simulink model "IEEE9_16b_forward"  (R2020a)
settings: Solver=VariableStepAuto  StartTime=0.0  StopTime=5  MaxStep=1e-4  RelTol=1e-3
libraries: powerlib x33, dspsigops x6, sps_avr x3
(part 1 of 2)
settings Model: Creator=Pankaj  LastModifiedBy=ahmed
settings DataIOCC: ReturnWorkspaceOutputs=off
settings DebuggingCC: UnconnectedInputMsg=none  UnconnectedOutputMsg=none  UnconnectedLineMsg=none  ArithmeticOperatorsInVariantConditions=warning
settings SFSimCC: SimUseLocalCustomCode=off  CustomCodeUndefinedFunction=UseInterfaceOnly
settings RTWCC: RTWUseLocalCustomCode=off
settings CodeAppCC: StateflowObjectComments=on
settings SimscapeCC: SimscapeNormalizeSystem=off

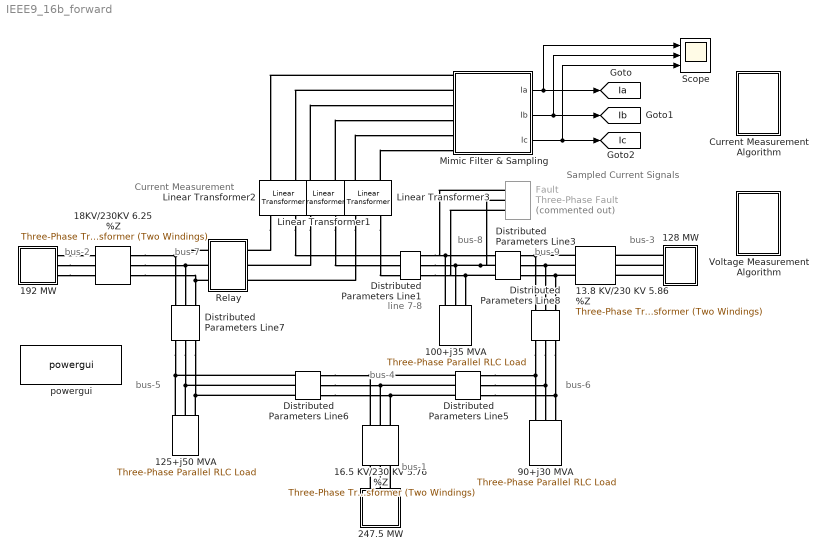
== system IEEE9_16b_forward ==
  note: Current Measurement
  note: Sampled Current Signals
  note: bus-2
  note: bus-7
  note: bus-8
  note: bus-9
  note: bus-1
  note: bus-3
  note: bus-4
  note: bus-6
  note: bus-5
  note: line 7-8
  100+j35 MVA : powerlib/Elements/Three-Phase Parallel RLC Load  LConnTagsString=A|B|C  Configuration=Y (grounded)  NominalVoltage=(230000)*0.993698  Vabc=[1e3 1e3 1e3]  Vabcp=[1e3 1e3 1e3]  NominalFrequency=60  UnbalancedPower=off  ActivePower=100e6  InductivePower=35e6  CapacitivePower=0  Pabc=[10e3 9e3 11e3]  QLabc=[100 90 110]  QCabc=[100 90 110]  Pabcp=[10e3 9e3 11e3]  QLabcp=[100 90 110]  QCabcp=[100 90 110]  Measurements=None  LoadType=constant PQ
  125+j50 MVA : powerlib/Elements/Three-Phase Parallel RLC Load  LConnTagsString=A|B|C  Configuration=Y (grounded)  NominalVoltage=(223027)*1  Vabc=[1e3 1e3 1e3]  Vabcp=[1e3 1e3 1e3]  NominalFrequency=60  UnbalancedPower=off  ActivePower=125e6  InductivePower=50e6  CapacitivePower=0  Pabc=[10e3 9e3 11e3]  QLabc=[100 90 110]  QCabc=[100 90 110]  Pabcp=[10e3 9e3 11e3]  QLabcp=[100 90 110]  QCabcp=[100 90 110]  Measurements=None  LoadType=constant PQ
  128 MW : Subsystem
  13.8 KV/230 KV 5.86 %Z : powerlib/Elements/Three-Phase Transformer (Two Windings)  Winding1Connection=Yg  Winding2Connection=Yg  CoreType=Three single-phase transformers  SetSaturation=off  Hysteresis=off  DataFile='hysteresis'  SetInitialFlux=off  Measurements=None  UNITS=pu  NominalPower=[ 100e6 , 60 ]  Winding1=[13.8e3 , 1e-6 , 0 ]  Winding2=[ 230e3 , 1e-6, 0.0586 ]  Rm=500  Lm=500  L0=0.5  Saturation=[ 0,0 ; 0.0024,1.2 ; 1.0,1.52 ]  InitialFluxes=[ 0.8 , -0.8 , 0.7 ]  BreakLoop=off  DiscreteSolver=Trapezoidal iterative  DataType=off  TransfoNumber=1
  "16.5 KV/230 KV 5.76 %Z     " : powerlib/Elements/Three-Phase Transformer (Two Windings)  Winding1Connection=Yg  Winding2Connection=Yg  CoreType=Three single-phase transformers  SetSaturation=off  Hysteresis=off  DataFile='hysteresis'  SetInitialFlux=off  Measurements=None  UNITS=pu  NominalPower=[ 100e6 , 60 ]  Winding1=[16.5e3 , 1e-6, 0 ]  Winding2=[ 230e3 ,1e-6, 0.0576 ]  Rm=500  Lm=500  L0=0.5  Saturation=[ 0,0 ; 0.0024,1.2 ; 1.0,1.52 ]  InitialFluxes=[ 0.8 , -0.8 , 0.7 ]  BreakLoop=off  DiscreteSolver=Trapezoidal iterative  DataType=off  TransfoNumber=1
  18KV/230KV 6.25 %Z : powerlib/Elements/Three-Phase Transformer (Two Windings)  Winding1Connection=Yg  Winding2Connection=Yg  CoreType=Three single-phase transformers  SetSaturation=off  Hysteresis=off  DataFile='hysteresis'  SetInitialFlux=off  Measurements=None  UNITS=pu  NominalPower=[ 100e6 , 60 ]  Winding1=[ 18e3 , 1e-6 , 0]  Winding2=[ 230e3 , 1e-6, 0.0625 ]  Rm=500  Lm=500  L0=0.5  Saturation=[ 0,0 ; 0.0024,1.2 ; 1.0,1.52 ]  InitialFluxes=[ 0.8 , -0.8 , 0.7 ]  BreakLoop=off  DiscreteSolver=Trapezoidal iterative  DataType=off  TransfoNumber=1
  192 MW : Subsystem
  247.5 MW : Subsystem
  90+j30 MVA : powerlib/Elements/Three-Phase Parallel RLC Load  LConnTagsString=A|B|C  Configuration=Y (grounded)  NominalVoltage=(226177)*0.999999  Vabc=[1e3 1e3 1e3]  Vabcp=[1e3 1e3 1e3]  NominalFrequency=60  UnbalancedPower=off  ActivePower=90e6  InductivePower=30e6  CapacitivePower=0  Pabc=[10e3 9e3 11e3]  QLabc=[100 90 110]  QCabc=[100 90 110]  Pabcp=[10e3 9e3 11e3]  QLabcp=[100 90 110]  QCabcp=[100 90 110]  Measurements=None  LoadType=constant PQ
  "Current Measurement Algorithm " : Subsystem
  Distributed Parameters Line1 : powerlib/Elements/Distributed Parameters Line  Phases=3  Frequency=60  Resistance=[0.044965 0.11241]  Inductance="[1.01e-3  2.02e-3]"  Capacitance=[12.74e-9 7.751e-9]  Length=100  x1=[-0.000416666666666667 3.75387602022078e-10 0 0;-0.000388888888888889 3.7197824084154e-10 0 0;-0.000361111111111111 3.68528088055081e-10 74821.3370893516 -218003.688402658;-0.000333333333333333 3.65037522010832e-10 77100.1170863376 -217208.220837109;-0.000305555555555556 3.61506925488695e-10 79370.4421866458 -216388.933942431;-0.000277777777777778 3.57936685658366e-10 81632.0634235446 -215545.917562665;-0.00025 3.54327194036874e-10 83884.7327847793 -214679.264144056;-0.000222222222222222 3.50678846445652e-10 86128.2032397691 -213789.068724919;-0.000194444444444444 3.46992042967126e-10 88362.228766697 -212875.428925212;-0.000166666666666667 3.43267187900843e-10 90586.5643794889 -211938.444935835;-0.000138888888888889 3.39504689719137e-10 92800.9661546787 -210978.219507642;-0.000111111111111111 3.35704961022334e-10 95005.1912581579 -209994.857940171;-8.33333333333333e-05 3.31868418493504e-10 97198.9979718044 -208988.468070101;-5.55555555555556e-05 3.27995482852768e-10 99382.1457199901 -207959.16025942;-2.77777777777778e-05 3.24086578811165e-10 101554.395095963 -206907.04738333]  x2=[-0.000416666666666667 2.64824658741118e-10 0 0;-0.000388888888888889 2.63860811791274e-10 0 0;-0.000361111111111111 2.62868029529975e-10 64739.8204195497 -219141.802960464;-0.000333333333333333 2.61846420826985e-10 67031.0711258709 -218451.845228193;-0.000305555555555556 2.6079609771321e-10 69314.9711198716 -217737.931789363;-0.000277777777777778 2.59717175368416e-10 71591.2699461803 -217000.14093263;-0.00025 2.58609772108597e-10 73859.7179829791 -216238.553565074;-0.000222222222222222 2.57474009372998e-10 76120.0664693777 -215453.253203332;-0.000194444444444444 2.56310011710804e-10 78372.0675326927 -214644.325964439;-0.000166666666666667 2.55117906767474e-10 80615.4742156299 -213811.860556383;-0.000138888888888889 2.53897825270749e-10 82850.0405033655 -212955.948268376;-0.000111111111111111 2.52649901016315e-10 85075.5213505248 -212076.682960845;-8.33333333333333e-05 2.51374270853129e-10 87291.6727080541 -211174.161055141;-5.55555555555556e-05 2.50071074668414e-10 89498.2515499831 -210248.481522961;-2.77777777777778e-05 2.48740455372316e-10 91695.0159000761 -209299.745875497]  x3=[-0.000416666666666667 -2.04003898439344e-12 0 0;-0.000388888888888889 -2.05746740304678e-12 0 0;-0.000361111111111111 -2.07467019721381e-12 150.649252870724 -526.476156782274;-0.000333333333333333 -2.09164548041432e-12 156.154138622374 -524.869725989955;-0.000305555555555556 -2.1083913911172e-12 161.641900313027 -523.205737317437;-0.000277777777777778 -2.12490609294463e-12 167.111936147772 -521.48437323983;-0.00025 -2.14118777487345e-12 172.563646275538 -519.705822524101;-0.000222222222222222 -2.15723465143376e-12 177.996432854874 -517.870280208381;-0.000194444444444444 -2.17304496290472e-12 183.40970011951 -515.977947580569;-0.000166666666666667 -2.18861697550751e-12 188.802854443689 -514.029032156261;-0.000138888888888889 -2.20394898159546e-12 194.175304407263 -512.023747655997;-0.000111111111111111 -2.21903929984133e-12 199.526460860552 -509.962313981818;-8.33333333333333e-05 -2.23388627542167e-12 204.855736988949 -507.844957193159;-5.55555555555556e-05 -2.2484882801983e-12 210.162548377271 -505.671909482051;-2.77777777777778e-05 -2.26284371289685e-12 215.446313073846 -503.443409147664]  x4=[-0.000416666666666667 4.10473658759201e-12 0 0;-0.000388888888888889 4.11161754213951e-12 0 0;-0.000361111111111111 4.1180476114898e-12 234.808229613019 -1040.8879000901;-0.000333333333333333 4.12402609051331e-12 245.695270450749 -1038.37195913634;-0.000305555555555556 4.12955232360244e-12 256.555368033339 -1035.74214899586;-0.000277777777777778 4.13462570474346e-12 267.387331428709 -1032.998758057;-0.00025 4.13924567758297e-12 278.189972790006 -1030.14208716347;-0.000222222222222222 4.14341173548886e-12 288.96210748587 -1027.17244958145;-0.000194444444444444 4.14712342160596e-12 299.702554230342 -1024.09017096514;-0.000166666666666667 4.15038032890604e-12 310.410135212401 -1020.89558932114;-0.000138888888888889 4.15318210023252e-12 321.083676225131 -1017.58905497133;-0.000111111111111111 4.1555284283396e-12 331.722006794478 -1014.17093051445;-8.33333333333333e-05 4.15741905592597e-12 342.323960307612 -1010.64159078637;-5.55555555555556e-05 4.158853775663e-12 352.888374140859 -1007.00142281896;-2.77777777777778e-05 4.15983243021751e-12 363.414089787191 -1003.25082579767]  x5=0.000395689524753941  V1=[5.416e-10 2.305e+05 2.305e+05;377 377 377;2.885 0.3359 -1.235]  V2=[2.789e-10 2.285e+05 2.285e+05;377 377 377;2.728 0.2916 -1.279]  I1=[3.179e-12 542 542;377 377 377;-1.76 0.2811 -1.29]  I2=[4.124e-12 1072 1072;377 377 377;1.614 0.2282 -1.343]  nHarmo=1  Measurements=None
  Distributed Parameters Line3 : powerlib/Elements/Distributed Parameters Line  Phases=3  Frequency=60  Resistance=[ 0.062951 0.15737]  Inductance="[ 1.414e-3  3.53e-3]"  Capacitance=[12.74e-9 7.751e-9]  Length=100  x1=[-0.000527777777777778 2.55561950726395e-10 0 0;-0.0005 2.54610764389849e-10 0 0;-0.000472222222222222 2.53631657113786e-10 0 0;-0.000444444444444444 2.52624736268351e-10 57824.4805062983 -221067.198486087;-0.000416666666666667 2.51590112273762e-10 60136.2726943207 -220449.551294082;-0.000388888888888889 2.50527898588199e-10 62441.4702623681 -219807.729324537;-0.000361111111111111 2.49438211695364e-10 64739.8204195497 -219141.802960464;-0.000333333333333333 2.48321171091703e-10 67031.0711258709 -218451.845228193;-0.000305555555555556 2.47176899273306e-10 69314.9711198716 -217737.931789363;-0.000277777777777778 2.46005521722474e-10 71591.2699461803 -217000.14093263;-0.00025 2.44807166893954e-10 73859.7179829791 -216238.553565074;-0.000222222222222222 2.43581966200859e-10 76120.0664693777 -215453.253203332;-0.000194444444444444 2.4233005400025e-10 78372.0675326928 -214644.325964439;-0.000166666666666667 2.41051567578409e-10 80615.4742156299 -213811.860556383;-0.000138888888888889 2.39746647135779e-10 82850.0405033655 -212955.948268376;-0.000111111111111111 2.38415435771591e-10 85075.5213505248 -212076.682960845;-8.33333333333333e-05 2.37058079468173e-10 87291.6727080541 -211174.161055141;-5.55555555555556e-05 2.35674727074939e-10 89498.2515499831 -210248.481522961;-2.77777777777778e-05 2.34265530292069e-10 91695.0159000761 -209299.745875497]  x2=[-0.000527777777777778 4.29111103751213e-11 0 0;-0.0005 4.22221066311759e-11 0 0;-0.000472222222222222 4.15284727574384e-11 0 0;-0.000444444444444444 4.08302848186798e-11 67173.7616448814 -221262.54243476;-0.000416666666666667 4.01276193790753e-11 69487.0865516397 -220546.981425706;-0.000388888888888889 3.94205534938088e-11 71792.7914163093 -219807.234954801;-0.000361111111111111 3.87091647006223e-11 74090.6233923689 -219043.384143581;-0.000333333333333333 3.79935310113139e-11 76380.3304966481 -218255.512756895;-0.000305555555555556 3.72737309031818e-11 78661.6616369602 -217443.707193719;-0.000277777777777778 3.65498433104194e-11 80934.3666396375 -216608.056477681;-0.00025 3.58219476154588e-11 83198.1962769654 -215748.6522473;-0.000222222222222222 3.50901236402655e-11 85452.902294513 -214865.588745933;-0.000194444444444444 3.43544516375852e-11 87698.2374383574 -213958.962811446;-0.000166666666666667 3.36150122821434e-11 89933.9554821973 -213028.873865587;-0.000138888888888889 3.28718866617982e-11 92159.811254355 -212075.423903092;-0.000111111111111111 3.21251562686479e-11 94375.560664662 -211098.717480494;-8.33333333333333e-05 3.13749029900952e-11 96580.9607312263 -210098.861704657;-5.55555555555556e-05 3.06212090998666e-11 98775.7696070778 -209075.966221035;-2.77777777777778e-05 2.98641572489906e-11 100959.74660669 -208030.143201645]  x3=[-0.000527777777777778 -2.39362255513196e-13 0 0;-0.0005 -2.59660907313448e-13 0 0;-0.000472222222222222 -2.799310843691e-13 0 0;-0.000444444444444444 -3.00170563826815e-13 135.04006780187 -840.518017098255;-0.000416666666666667 -3.20377126199591e-13 143.834380612161 -839.057826267368;-0.000388888888888889 -3.40548555610158e-13 152.612920361752 -837.505623290508;-0.000361111111111111 -3.60682640033968e-13 161.374724384834 -835.861578384224;-0.000333333333333333 -3.80777171541775e-13 170.11883185086 -834.125871836566;-0.000305555555555556 -4.00829946541753e-13 178.844283869907 -832.298693987316;-0.000277777777777778 -4.2083876602115e-13 187.550123597837 -830.380245207118;-0.00025 -4.40801435787432e-13 196.235396341216 -828.370735875497;-0.000222222222222222 -4.60715766708898e-13 204.899149662015 -826.270386357799;-0.000194444444444444 -4.8057957495475e-13 213.540433482049 -824.079426981015;-0.000166666666666667 -5.00390682234569e-13 222.158300187171 -821.798098008531;-0.000138888888888889 -5.2014691603719e-13 230.75180473118 -819.426649613778;-0.000111111111111111 -5.39846109868945e-13 239.320004739464 -816.965341852796;-8.33333333333333e-05 -5.59486103491239e-13 247.861960612337 -814.414444635717;-5.55555555555556e-05 -5.79064743157451e-13 256.376735628079 -811.774237697167;-2.77777777777778e-05 -5.98579881849109e-13 264.863396045655 -809.04501056559]  x4=[-0.000527777777777778 1.05597372399963e-12 0 0;-0.0005 1.06804867740089e-12 0 0;-0.000472222222222222 1.08000650722885e-12 0 0;-0.000444444444444444 1.09184590217273e-12 129.425410784576 -498.290871237006;-0.000416666666666667 1.10356556390945e-12 134.636282980495 -496.908230379704;-0.000388888888888889 1.11516420724603e-12 139.832390790773 -495.471097935293;-0.000361111111111111 1.12664056026053e-12 145.013164403632 -493.979631501542;-0.000333333333333333 1.13799336444152e-12 150.178035688865 -492.433994634553;-0.000305555555555556 1.14922137482607e-12 155.326438260132 -490.834356830825;-0.000277777777777778 1.16032336013632e-12 160.457807537074 -489.18089350867;-0.00025 1.17129810291448e-12 165.571580807224 -487.473785988975;-0.000222222222222222 1.18214439965633e-12 170.667197287716 -485.713221475315;-0.000194444444444444 1.1928610609432e-12 175.744098186782 -483.89939303343;-0.000166666666666667 1.20344691157241e-12 180.801726765025 -482.032499570049;-0.000138888888888889 1.21390079068615e-12 185.839528396478 -480.112745811077;-0.000111111111111111 1.22422155189878e-12 190.856950629422 -478.140342279148;-8.33333333333333e-05 1.23440806342252e-12 195.853443246966 -476.115505270536;-5.55555555555556e-05 1.24445920819159e-12 200.828458327391 -474.038456831437;-2.77777777777778e-05 1.2543738839847e-12 205.781450304229 -471.909424733619]  x5=0.000523077718890797  V1=[2.541e-10 2.285e+05 2.285e+05;377 377 377;2.713 0.2668 -1.304]  V2=[4.31e-10 2.313e+05 2.313e+05;377 377 377;2.564 0.3044 -1.266]  I1=[1.418e-12 846 846;377 377 377;1.513 0.1676 -1.403]  I2=[2.062e-12 520.4 520.5;377 377 377;-2.991 0.2668 -1.304]  nHarmo=1  Measurements=None
  Distributed Parameters Line5 : powerlib/Elements/Distributed Parameters Line  Phases=3  Frequency=60  Resistance=[ 0.08993 0.224825]  Inductance="[ 1.29e-3  3.22e-3]"  Capacitance=[12.74e-9 7.751e-9]  Length=100  x1=[-0.0005 1.66779418345913e-10 59546.3118778118 -220996.591907279;-0.000472222222222222 1.66560469061081e-10 61857.2703455525 -220360.917131056;-0.000444444444444444 1.6632325454385e-10 64161.4454665317 -219701.077297027;-0.000416666666666667 1.66067800807466e-10 66458.5845619817 -219017.144764067;-0.000388888888888889 1.65794135865309e-10 68748.4357247144 -218309.194533084;-0.000361111111111111 1.65502289727824e-10 71030.7478467454 -217577.3042388;-0.000333333333333333 1.6519229439923e-10 73305.2706468312 -216821.554141233;-0.000305555555555556 1.64864183874006e-10 75571.7546979152 -216042.027116897;-0.000277777777777778 1.6451799413317e-10 77829.9514544804 -215238.808649716;-0.00025 1.64153763140329e-10 80079.6132798047 -214411.986821645;-0.000222222222222222 1.63771530837514e-10 82320.4934731177 -213561.652303016;-0.000194444444444444 1.63371339140806e-10 84552.3462966537 -212687.89834259;-0.000166666666666667 1.62953231935733e-10 86774.9270026 -211790.820757337;-0.000138888888888889 1.62517255072462e-10 88987.9918599359 -210870.517921922;-0.000111111111111111 1.62063456360769e-10 91191.2981811608 -209927.090757922;-8.33333333333333e-05 1.61591885564798e-10 93384.6043489076 -208960.642722757;-5.55555555555556e-05 1.61102594397599e-10 95567.6698424387 -207971.279798346;-2.77777777777778e-05 1.60595636515463e-10 97740.2552640219 -206959.110479481]  x2=[-0.0005 4.01983523522078e-11 47854.5977364337 -220989.473150866;-0.000472222222222222 3.88026912842948e-11 50166.1226469457 -220476.232676798;-0.000444444444444444 3.74027750640158e-11 52472.1462767887 -219938.814499276;-0.000416666666666667 3.59987572079602e-11 54772.4157444851 -219377.277552259;-0.000388888888888889 3.45907916825075e-11 57066.678799566 -218791.683414601;-0.000361111111111111 3.31790328869441e-11 59354.6838502336 -218182.096303299;-0.000333333333333333 3.17636356365309e-11 61636.1799909505 -217548.583066448;-0.000305555555555556 3.03447551455266e-11 63910.9170299547 -216891.213175914;-0.000277777777777778 2.89225470101662e-11 66178.6455166961 -216210.058719714;-0.00025 2.74971671915987e-11 68439.116769191 -215505.194394109;-0.000222222222222222 2.60687719987837e-11 70692.0829012934 -214776.697495416;-0.000194444444444444 2.46375180713506e-11 72937.2968498783 -214024.647911529;-0.000166666666666667 2.32035623624215e-11 75174.512401935 -213249.12811316;-0.000138888888888889 2.17670621213989e-11 77403.4842215671 -212450.223144794;-0.000111111111111111 2.03281748767223e-11 79623.9678768963 -211628.020615364;-8.33333333333333e-05 1.88870584185926e-11 81835.7198668672 -210782.610688643;-5.55555555555556e-05 1.74438707816696e-11 84038.49764795 -209914.086073355;-2.77777777777778e-05 1.59987702277409e-11 86232.0596607379 -209022.542013013]  x3=[-0.0005 8.71928217285157e-13 88.5714316521851 -463.888694962859;-0.000472222222222222 8.53672647821716e-13 93.4243168618632 -462.935760457911;-0.000444444444444444 8.35323463532424e-13 98.2669570424012 -461.932059830018;-0.000416666666666667 8.16882676612116e-13 103.098821143731 -460.877703146263;-0.000388888888888889 7.98352309300887e-13 107.919379297505 -459.772806028739;-0.000361111111111111 7.7973439366233e-13 112.728102875198 -458.617489641864;-0.000333333333333333 7.610309713607e-13 117.524464546081 -457.411880679102;-0.000305555555555556 7.42244093437021e-13 122.307938335045 -456.156111349059;-0.000277777777777778 7.23375820084165e-13 127.077999680286 -454.850319360995;-0.00025 7.04428220420933e-13 131.834125490823 -453.494647909716;-0.000222222222222222 6.85403372265147e-13 136.575794203865 -452.089245659873;-0.000194444444444444 6.66303361905799e-13 141.302485842002 -450.634266729661;-0.000166666666666667 6.47130283874261e-13 146.013682070233 -449.129870673915;-0.000138888888888889 6.278862407146e-13 150.7088662528 -447.576222466616;-0.000111111111111111 6.08573342753011e-13 155.387523509849 -445.973492482799;-8.33333333333333e-05 5.8919370786639e-13 160.049140773886 -444.321856479866;-5.55555555555556e-05 5.69749461250093e-13 164.693206846047 -442.621495578318;-2.77777777777778e-05 5.50242735184876e-13 169.319212452153 -440.872596241888]  x4=[-0.0005 -5.67274624614988e-13 137.008206439645 -921.42394011898;-0.000472222222222222 -5.57955314738249e-13 146.649614941233 -919.938692916882;-0.000444444444444444 -5.48574818773665e-13 156.274941659952 -918.352564070339;-0.000416666666666667 -5.39134165398325e-13 165.88313107026 -916.665727516253;-0.000388888888888889 -5.2963438988626e-13 175.473129525912 -914.878368235261;-0.000361111111111111 -5.20076533994906e-13 185.04388537551 -912.99068223145;-0.000333333333333333 -5.1046164585087e-13 194.594349077822 -911.002876510862;-0.000305555555555556 -5.00790779834987e-13 204.123473316877 -908.915169058795;-0.000277777777777778 -4.91064996466696e-13 213.630213116822 -906.727788815899;-0.00025 -4.81285362287742e-13 223.113525956504 -904.440975653065;-0.000222222222222222 -4.71452949745221e-13 232.572371883804 -902.054980345127;-0.000194444444444444 -4.61568837073968e-13 242.005713629675 -899.570064543359;-0.000166666666666667 -4.51634108178322e-13 251.41251672189 -896.986500746781;-0.000138888888888889 -4.41649852513261e-13 260.791749598484 -894.304572272276;-0.000111111111111111 -4.3161716496493e-13 270.142383720879 -891.524573223525;-8.33333333333333e-05 -4.21537145730577e-13 279.463393686672 -888.646808458752;-5.55555555555556e-05 -4.11410900197903e-13 288.75375734208 -885.671593557291;-2.77777777777778e-05 -4.01239538823842e-13 298.012455894037 -882.599254784986]  x5=0.000499582025297148  V1=[3.29e-10 2.289e+05 2.289e+05;377 377 377;2.341 0.2974 -1.273]  V2=[3.35e-10 2.261e+05 2.261e+05;377 377 377;2.353 0.2487 -1.322]  I1=[9.5e-13 477.9 477.9;377 377 377;2.529 0.2254 -1.345]  I2=[6.245e-14 926.2 926.2;377 377 377;-2.223 0.1812 -1.39]  nHarmo=1  Measurements=None
  Distributed Parameters Line6 : powerlib/Elements/Distributed Parameters Line  Phases=3  Frequency=60  Resistance=[ 0.0529 0.13225]  Inductance="[ 1.192e-3  2.38e-3]"  Capacitance=[12.74e-9 7.751e-9]  Length=100  x1=[-0.000444444444444444 4.40363838311251e-10 0 0;-0.000416666666666667 4.3957416386782e-10 51582.9063755373 -216854.565020272;-0.000388888888888889 4.3873628516377e-10 53850.9272011653 -216302.50863973;-0.000361111111111111 4.37850294081944e-10 56113.042665781 -215726.732251609;-0.000333333333333333 4.36916287781247e-10 58369.0047029318 -215127.298996277;-0.000305555555555556 4.35934368685996e-10 60618.565920958 -214504.274608346;-0.000277777777777778 4.34904644474685e-10 62861.4796301218 -213857.72740946;-0.00025 4.33827228068177e-10 65097.4998696597 -213187.728300807;-0.000222222222222222 4.32702237617323e-10 67326.3814347548 -212494.350755338;-0.000194444444444444 4.31529796490003e-10 69547.8799034262 -211777.670809715;-0.000166666666666667 4.303100332576e-10 71761.7516633328 -211037.76705597;-0.000138888888888889 4.29043081680896e-10 73967.7539384881 -210274.720632888;-0.000111111111111111 4.2772908069541e-10 76165.6448158832 -209488.615217108;-8.33333333333333e-05 4.26368174396157e-10 78355.1832720154 -208679.537013947;-5.55555555555556e-05 4.24960512021849e-10 80536.1291993192 -207847.574747948;-2.77777777777778e-05 4.23506247938528e-10 82708.2434324966 -206992.819653149]  x2=[-0.000444444444444444 1.6632325454385e-10 0 0;-0.000416666666666667 1.66067800807466e-10 66458.5845619817 -219017.144764067;-0.000388888888888889 1.65794135865309e-10 68748.4357247144 -218309.194533084;-0.000361111111111111 1.65502289727824e-10 71030.7478467454 -217577.3042388;-0.000333333333333333 1.6519229439923e-10 73305.2706468312 -216821.554141233;-0.000305555555555556 1.64864183874006e-10 75571.7546979152 -216042.027116897;-0.000277777777777778 1.6451799413317e-10 77829.9514544804 -215238.808649716;-0.00025 1.64153763140329e-10 80079.6132798047 -214411.986821645;-0.000222222222222222 1.63771530837514e-10 82320.4934731177 -213561.652303016;-0.000194444444444444 1.63371339140806e-10 84552.3462966537 -212687.89834259;-0.000166666666666667 1.62953231935733e-10 86774.9270026 -211790.820757337;-0.000138888888888889 1.62517255072462e-10 88987.9918599359 -210870.517921922;-0.000111111111111111 1.62063456360769e-10 91191.2981811608 -209927.090757922;-8.33333333333333e-05 1.61591885564798e-10 93384.6043489076 -208960.642722757;-5.55555555555556e-05 1.61102594397599e-10 95567.6698424387 -207971.279798346;-2.77777777777778e-05 1.60595636515463e-10 97740.2552640219 -206959.110479481]  x3=[-0.000444444444444444 -5.75359111964091e-13 0 0;-0.000416666666666667 -6.03191143182178e-13 105.580871188103 -1042.52650014874;-0.000388888888888889 -6.30957027694068e-13 116.492169433156 -1041.36371643476;-0.000361111111111111 -6.58653720657633e-13 127.390692999084 -1040.08673545418;-0.000333333333333333 -6.86278184818375e-13 138.275246739962 -1038.69569724233;-0.000305555555555556 -7.13827390842499e-13 149.144637041814 -1037.19075434225;-0.000277777777777778 -7.41298317649113e-13 159.997671953507 -1035.57207178788;-0.00025 -7.68687952741525e-13 170.833161317461 -1033.839827086;-0.000222222222222222 -7.95993292537593e-13 181.649916900162 -1031.99421019677;-0.000194444444444444 -8.23211342699104e-13 192.446752522466 -1030.03542351287;-0.000166666666666667 -8.50339118460141e-13 203.222484189678 -1027.96368183733;-0.000138888888888889 -8.77373644954387e-13 213.975930221389 -1025.77921235999;-0.000111111111111111 -9.04311957541361e-13 224.705911381062 -1023.48225463253;-8.33333333333333e-05 -9.31151102131522e-13 235.411251005347 -1021.07306054225;-5.55555555555556e-05 -9.57888135510215e-13 246.090775133116 -1018.55189428443;-2.77777777777778e-05 -9.84520125660431e-13 256.7433126342 -1015.91903233337]  x4=[-0.000444444444444444 5.85836689934932e-13 0 0;-0.000416666666666667 6.18309927099945e-13 171.38904947301 -392.212001612646;-0.000388888888888889 6.50715359613731e-13 175.48680323776 -390.395742913017;-0.000361111111111111 6.8304943385544e-13 179.565312896977 -388.536672920819;-0.000333333333333333 7.15308604029459e-13 183.624131196119 -386.634995504024;-0.000305555555555556 7.47489332554251e-13 187.662813040019 -384.690919202992;-0.000277777777777778 7.7958809045029e-13 191.680915541702 -382.704657207596;-0.00025 8.11601357727051e-13 195.677998070947 -380.676427333848;-0.000222222222222222 8.43525623769022e-13 199.653622302614 -378.60645200001;-0.000194444444444444 8.75357387720676e-13 203.607352264703 -376.494958202203;-0.000166666666666667 9.07093158870386e-13 207.538754386171 -374.342177489516;-0.000138888888888889 9.38729457033215e-13 211.44739754447 -372.148345938615;-0.000111111111111111 9.7026281293256e-13 215.332853112833 -369.913704127851;-8.33333333333333e-05 1.0016897685806e-12 219.194695007272 -367.638497110881;-5.55555555555556e-05 1.0330068776575e-12 223.032499733304 -365.322974389793;-2.77777777777778e-05 1.06421070588933e-12 226.845846432391 -362.967389887748]  x5=0.000429504132692574  V1=[5.692e-10 2.23e+05 2.23e+05;377 377 377;2.022 0.2411 -1.33]  V2=[3.29e-10 2.289e+05 2.289e+05;377 377 377;2.367 0.3033 -1.267]  I1=[3.839e-12 1053 1053;377 377 377;3.112 0.1114 -1.459]  I2=[2.337e-12 422.3 422.3;377 377 377;0.2722 0.4185 -1.152]  nHarmo=1  Measurements=None
  Distributed Parameters Line7 : powerlib/Elements/Distributed Parameters Line  Phases=3  Frequency=60  Resistance=[ 0.16928 0.4232]  Inductance="[ 2.259e-3  5.64e-3]"  Capacitance=[12.74e-9 7.751e-9]  Length=100  x1=[-0.000666666666666667 4.41317688924231e-10 30946.2075590005 -220746.546513486;-0.000638888888888889 4.41064115665892e-10 33256.1158216911 -220410.380267001;-0.000611111111111111 4.40762174756929e-10 35562.3771765195 -220050.043538521;-0.000583333333333333 4.40411899308566e-10 37864.7387159389 -219665.575843028;-0.000555555555555556 4.40013327732452e-10 40162.9479600613 -219257.019341738;-0.000527777777777778 4.39566503736453e-10 42456.7528843446 -218824.418837476;-0.0005 4.39071476319856e-10 44745.90194723 -218367.82176976;-0.000472222222222222 4.38528299767993e-10 47030.1441177263 -217887.278209606;-0.000444444444444445 4.37937033646297e-10 49309.2289029387 -217382.84085403;-0.000416666666666667 4.3729774279376e-10 51582.9063755373 -216854.565020272;-0.000388888888888889 4.36610497315827e-10 53850.9272011653 -216302.50863973;-0.000361111111111111 4.35875372576711e-10 56113.0426657809 -215726.732251609;-0.000333333333333333 4.35092449191122e-10 58369.0047029318 -215127.298996277;-0.000305555555555556 4.34261813015434e-10 60618.565920958 -214504.274608346;-0.000277777777777778 4.33383555138263e-10 62861.4796301218 -213857.72740946;-0.00025 4.32457771870481e-10 65097.4998696597 -213187.728300807;-0.000222222222222222 4.31484564734659e-10 67326.3814347548 -212494.350755338;-0.000194444444444444 4.30464040453924e-10 69547.8799034262 -211777.670809715;-0.000166666666666667 4.29396310940264e-10 71761.7516633328 -211037.76705597;-0.000138888888888889 4.28281493282253e-10 73967.7539384881 -210274.720632888;-0.000111111111111111 4.2711970973221e-10 76165.6448158832 -209488.615217108;-8.33333333333333e-05 4.25911087692793e-10 78355.1832720154 -208679.537013947;-5.55555555555556e-05 4.24655759703029e-10 80536.1291993192 -207847.574747948;-2.77777777777778e-05 4.23353863423778e-10 82708.2434324966 -206992.819653149]  x2=[-0.000666666666666667 3.89319476015602e-10 51304.2793847977 -224516.169341558;-0.000638888888888889 3.8751300125057e-10 53652.5460449753 -223966.61067393;-0.000611111111111111 3.85664031318076e-10 55994.92909887 -223392.491543567;-0.000583333333333333 3.83772768978509e-10 58331.1716777834 -222793.874909101;-0.000555555555555556 3.81839421630098e-10 60661.0175863898 -222170.826415594;-0.000527777777777778 3.79864201286166e-10 62984.2113308303 -221523.414387332;-0.0005 3.77847324551882e-10 65300.4981467308 -220851.70982034;-0.000472222222222222 3.75789012600509e-10 67609.6240271398 -220155.786374595;-0.000444444444444445 3.73689491149147e-10 69911.335750383 -219435.720365943;-0.000416666666666667 3.71548990433982e-10 72205.3809078321 -218691.590757737;-0.000388888888888889 3.6936774518504e-10 74491.5079315839 -217923.479152174;-0.000361111111111111 3.67145994600442e-10 76769.466122048 -217131.469781348;-0.000333333333333333 3.64883982320177e-10 79039.0056754386 -216315.649498011;-0.000305555555555556 3.62581956399382e-10 81299.8777111683 -215476.107766051;-0.000277777777777778 3.60240169281141e-10 83551.8342991405 -214612.936650679;-0.00025 3.578588777688e-10 85794.6284869383 -213726.230808335;-0.000222222222222222 3.55438342997808e-10 88028.0143269049 -212816.087476308;-0.000194444444444444 3.52978830407081e-10 90251.746903115 -211882.606462069;-0.000166666666666667 3.5048060970989e-10 92465.5823582324 -210925.890132333;-0.000138888888888889 3.47943954864287e-10 94669.2779202518 -209946.043401824;-0.000111111111111111 3.45369144043061e-10 96862.5919291215 -208943.173721779;-8.33333333333333e-05 3.42756459603234e-10 99045.283863244 -207917.39106816;-5.55555555555556e-05 3.40106188055097e-10 101217.114365852 -206868.807929595;-2.77777777777778e-05 3.37418620030792e-10 103377.845271256 -205797.539295041]  x3=[-0.000666666666666667 1.20662777610517e-12 21.8609357538281 -751.236078710436;-0.000638888888888889 1.20171260117632e-12 29.7265027167099 -750.965964353444;-0.000611111111111111 1.19666564491868e-12 37.5888098335816 -750.613498115843;-0.000583333333333333 1.19148746078787e-12 45.4469949138676 -750.178718649529;-0.000555555555555556 1.18617861663015e-12 53.3001962190203 -749.661673632969;-0.000527777777777778 1.1807396946201e-12 61.1475525570189 -749.062419765977;-0.0005 1.17517129119681e-12 68.9882033768093 -748.38102276349;-0.000472222222222222 1.16947401699846e-12 76.8212888626731 -747.61755734837;-0.000444444444444445 1.16364849679537e-12 84.6459500285158 -746.772107243203;-0.000416666666666667 1.15769536942148e-12 92.4613288120648 -745.844765161119;-0.000388888888888889 1.15161528770429e-12 100.266568168965 -744.835632795629;-0.000361111111111111 1.14540891839328e-12 108.060812166764 -743.744820809469;-0.000333333333333333 1.13907694208678e-12 115.843206078774 -742.572448822464;-0.000305555555555556 1.13262005315736e-12 123.612896477804 -741.318645398415;-0.000277777777777778 1.12603895967563e-12 131.369031329744 -739.983548030996;-0.00025 1.11933438333268e-12 139.110760087004 -738.567303128679;-0.000222222222222222 1.11250705936084e-12 146.837233781785 -737.070065998677;-0.000194444444444444 1.10555773645312e-12 154.547605119176 -735.492000829914;-0.000166666666666667 1.0984871766811e-12 162.241028570073 -733.833280675018;-0.000138888888888889 1.09129615541133e-12 169.916660463897 -732.094087431346;-0.000111111111111111 1.08398546122033e-12 177.573659081115 -730.274611821037;-8.33333333333333e-05 1.0765558958081e-12 185.21118474554 -728.375053370095;-5.55555555555556e-05 1.06900827391021e-12 192.828399916419 -726.395620386511;-2.77777777777778e-05 1.06134342320846e-12 200.424469280267 -724.336529937416]  x4=[-0.000666666666666667 -8.47360882882362e-14 62.4982199265413 -294.13588744843;-0.000638888888888889 -8.36103932599431e-14 65.5749130313703 -293.465291420381;-0.000611111111111111 -8.24755294098256e-14 68.6444151080233 -292.762513616075;-0.000583333333333333 -8.13316211884935e-14 71.7063895510074 -292.027631103018;-0.000555555555555556 -8.01787940383741e-14 74.7605005803197 -291.260724469357;-0.000527777777777778 -7.90171743799554e-14 77.8064132782691 -290.461877815049;-0.0005 -7.78468895979234e-14 80.843793626204 -289.63117874263;-0.000472222222222222 -7.66680680271923e-14 83.8723085411409 -288.768718347615;-0.000444444444444445 -7.54808389388314e-14 86.8916259122914 -287.874591208506;-0.000416666666666667 -7.42853325258891e-14 89.9014146374809 -286.948895376419;-0.000388888888888889 -7.30816798891157e-14 92.9013446594586 -285.991732364334;-0.000361111111111111 -7.18700130225868e-14 95.8910870020914 -285.003207135962;-0.000333333333333333 -7.06504647992285e-14 98.8703138064401 -283.983428094232;-0.000305555555555556 -6.94231689562467e-14 101.838698366713 -282.93250706941;-0.000277777777777778 -6.81882600804608e-14 104.795915166092 -281.850559306828;-0.00025 -6.69458735935452e-14 107.74163991243 -280.737703454251;-0.000222222222222222 -6.56961457371786e-14 110.675549573814 -279.594061548864;-0.000194444444444444 -6.44392135581037e-14 113.597322413987 -278.419759003889;-0.000166666666666667 -6.31752148930982e-14 116.506638027632 -277.214924594834;-0.000138888888888889 -6.19042883538598e-14 119.403177375507 -275.979690445368;-0.000111111111111111 -6.06265733118054e-14 122.286622819431 -274.714192012838;-8.33333333333333e-05 -5.93422098827879e-14 125.156658157118 -273.418568073405;-5.55555555555556e-05 -5.80513389117309e-14 128.01296865685 -272.092960706836;-2.77777777777778e-05 -5.67541019571832e-14 130.855241091995 -270.737515280916]  x5=0.000661178039562719  V1=[5.692e-10 2.23e+05 2.23e+05;377 377 377;1.934 0.1858 -1.385]  V2=[7.107e-10 2.305e+05 2.305e+05;377 377 377;2.15 0.2689 -1.302]  I1=[1.362e-12 746.7 746.7;377 377 377;1.537 0.07174 -1.499]  I2=[6.286e-13 306.4 306.4;377 377 377;-2.668 0.2582 -1.313]  nHarmo=1  Measurements=None
  Distributed Parameters Line8 : powerlib/Elements/Distributed Parameters Line  Phases=3  Frequency=60  Resistance=[ 0.20631 0.5157]  Inductance="[ 2.38e-3  6.09e-3]"  Capacitance=[12.74e-9 7.751e-9]  Length=100  x1=[-0.000694444444444444 4.98360423773267e-11 0 0;-0.000666666666666667 4.84744245360307e-11 0 0;-0.000638888888888889 4.71074909278272e-11 0 0;-0.000611111111111111 4.57353914523903e-11 0 0;-0.000583333333333333 4.43582765758896e-11 0 0;-0.000555555555555556 4.29762973144901e-11 43216.0585879023 -221943.198515761;-0.000527777777777778 4.15896052177911e-11 45537.8250300076 -221478.479638878;-0.0005 4.01983523522078e-11 47854.5977364337 -220989.473150866;-0.000472222222222222 3.88026912842948e-11 50166.1226469457 -220476.232676798;-0.000444444444444444 3.74027750640158e-11 52472.1462767887 -219938.814499276;-0.000416666666666667 3.59987572079602e-11 54772.415744485 -219377.277552259;-0.000388888888888889 3.45907916825075e-11 57066.678799566 -218791.683414601;-0.000361111111111111 3.31790328869441e-11 59354.6838502336 -218182.096303299;-0.000333333333333333 3.17636356365309e-11 61636.1799909505 -217548.583066448;-0.000305555555555556 3.03447551455266e-11 63910.9170299547 -216891.213175914;-0.000277777777777778 2.89225470101662e-11 66178.6455166961 -216210.058719714;-0.00025 2.74971671915987e-11 68439.116769191 -215505.194394109;-0.000222222222222222 2.60687719987837e-11 70692.0829012934 -214776.697495416;-0.000194444444444444 2.46375180713506e-11 72937.2968498783 -214024.647911529;-0.000166666666666667 2.32035623624215e-11 75174.512401935 -213249.12811316;-0.000138888888888889 2.17670621213989e-11 77403.4842215671 -212450.223144794;-0.000111111111111111 2.03281748767223e-11 79623.9678768963 -211628.020615364;-8.33333333333333e-05 1.88870584185926e-11 81835.7198668672 -210782.610688643;-5.55555555555556e-05 1.74438707816696e-11 84038.49764795 -209914.086073355;-2.77777777777778e-05 1.59987702277409e-11 86232.0596607379 -209022.542013013]  x2=[-0.000694444444444444 4.69437055011911e-11 0 0;-0.000666666666666667 4.62840508856103e-11 0 0;-0.000638888888888889 4.5619320702276e-11 0 0;-0.000611111111111111 4.49495878463436e-11 0 0;-0.000583333333333333 4.42749257615681e-11 0 0;-0.000555555555555556 4.35954084322498e-11 57849.3471893919 -223881.402427676;-0.000527777777777778 4.29111103751213e-11 60190.6075046368 -223263.341309905;-0.0005 4.22221066311759e-11 62525.2672414824 -222620.79685081;-0.000472222222222222 4.15284727574384e-11 64853.0703781792 -221953.839512632;-0.000444444444444444 4.08302848186798e-11 67173.7616448814 -221262.54243476;-0.000416666666666667 4.01276193790753e-11 69487.0865516397 -220546.981425706;-0.000388888888888889 3.94205534938088e-11 71792.7914163093 -219807.234954801;-0.000361111111111111 3.87091647006223e-11 74090.6233923689 -219043.384143581;-0.000333333333333333 3.79935310113139e-11 76380.3304966481 -218255.512756895;-0.000305555555555556 3.72737309031818e-11 78661.6616369603 -217443.707193719;-0.000277777777777778 3.65498433104194e-11 80934.3666396375 -216608.056477681;-0.00025 3.58219476154588e-11 83198.1962769654 -215748.6522473;-0.000222222222222222 3.50901236402655e-11 85452.902294513 -214865.588745933;-0.000194444444444444 3.43544516375852e-11 87698.2374383574 -213958.962811446;-0.000166666666666667 3.36150122821434e-11 89933.9554821973 -213028.873865587;-0.000138888888888889 3.28718866617982e-11 92159.811254355 -212075.423903092;-0.000111111111111111 3.21251562686479e-11 94375.560664662 -211098.717480494;-8.33333333333333e-05 3.13749029900952e-11 96580.9607312263 -210098.861704657;-5.55555555555556e-05 3.06212090998666e-11 98775.7696070778 -209075.966221035;-2.77777777777778e-05 2.98641572489906e-11 100959.74660669 -208030.143201645]  x3=[-0.000694444444444444 -1.45706326195069e-13 0 0;-0.000666666666666667 -1.46705756063926e-13 0 0;-0.000638888888888889 -1.47689097993406e-13 0 0;-0.000611111111111111 -1.48656244148987e-13 0 0;-0.000583333333333333 -1.49607088472193e-13 0 0;-0.000555555555555556 -1.5054152669223e-13 58.764642962532 -662.595775208533;-0.000527777777777778 -1.51459456337416e-13 65.699975413045 -661.94407841205;-0.0005 -1.52360776746422e-13 72.6281031208826 -661.219791987936;-0.000472222222222222 -1.53245389079307e-13 79.5482663387686 -660.422995362362;-0.000444444444444444 -1.54113196328362e-13 86.4597061928231 -659.553775913055;-0.000416666666666667 -1.54964103328741e-13 93.3616647657813 -658.612228959724;-0.000388888888888889 -1.55798016768903e-13 100.253385180107 -657.598457753603;-0.000361111111111111 -1.56614845200843e-13 107.134111680996 -656.512573466127;-0.000333333333333333 -1.57414499050117e-13 114.003089719247 -655.354695176747;-0.000305555555555556 -1.58196890625671e-13 120.859566034012 -654.124949859864;-0.000277777777777778 -1.5896193412945e-13 127.702788735397 -652.823472370911;-0.00025 -1.59709545665814e-13 134.532007386919 -651.450405431561;-0.000222222222222222 -1.60439643250733e-13 141.346473087792 -650.005899614077;-0.000194444444444444 -1.61152146820778e-13 148.145438555062 -648.490113324799;-0.000166666666666667 -1.61846978241906e-13 154.928158205546 -646.903212786775;-0.000138888888888889 -1.62524061318019e-13 161.693888237602 -645.245372021533;-0.000111111111111111 -1.63183321799329e-13 168.441886712688 -643.516772829995;-8.33333333333333e-05 -1.63824687390495e-13 175.171413636728 -641.71760477254;-5.55555555555556e-05 -1.64448087758552e-13 181.88173104126 -639.848065148222;-2.77777777777778e-05 -1.65053454540625e-13 188.572103064363 -637.908358973129]  x4=[-0.000694444444444444 1.53107988200119e-13 0 0;-0.000666666666666667 1.51583812326816e-13 0 0;-0.000638888888888889 1.50043013580298e-13 0 0;-0.000611111111111111 1.4848576092651e-13 0 0;-0.000583333333333333 1.46912225135753e-13 0 0;-0.000555555555555556 1.4532257876396e-13 61.9143778014845 -356.331561839114;-0.000527777777777778 1.4371699613377e-13 65.6423915716786 -355.663667992312;-0.0005 1.42095653315409e-13 69.3632069139144 -354.956771616349;-0.000472222222222222 1.4045872810739e-13 73.0764157988598 -354.21095023038;-0.000444444444444444 1.38806400017008e-13 76.7816110313165 -353.426285622123;-0.000416666666666667 1.37138850240659e-13 80.4783862948736 -352.602863838895;-0.000388888888888889 1.35456261643966e-13 84.1663361964643 -351.740775178175;-0.000361111111111111 1.3375881874173e-13 87.8450563108228 -350.840114177698;-0.000333333333333333 1.32046707677695e-13 91.5141432248329 -349.900979605092;-0.000305555555555556 1.30320116204131e-13 95.1731945817678 -348.923474447047;-0.000277777777777778 1.28579233661252e-13 98.8218091254124 -347.907705898019;-0.00025 1.26824250956445e-13 102.459586744066 -346.853785348476;-0.000222222222222222 1.25055360543342e-13 106.086128514418 -345.761828372682;-0.000194444444444444 1.23272756400709e-13 109.701036745297 -344.631954716026;-0.000166666666666667 1.21476634011179e-13 113.303915021278 -343.464288281886;-0.000138888888888889 1.19667190339813e-13 116.894368246158 -342.258957118045;-0.000111111111111111 1.17844623812499e-13 120.47200268628 -341.016093402648;-8.33333333333333e-05 1.16009134294196e-13 124.036426013712 -339.735833429708;-5.55555555555556e-05 1.14160923067013e-13 127.587247349268 -338.418317594157;-2.77777777777778e-05 1.12300192808139e-13 131.124077305374 -337.063690376454]  x5=0.000687048688231045  V1=[3.258e-10 2.261e+05 2.261e+05;377 377 377;2.369 0.194 -1.377]  V2=[4.31e-10 2.313e+05 2.313e+05;377 377 377;2.502 0.2568 -1.314]  I1=[9.177e-13 670.6 670.6;377 377 377;2.076 0.09296 -1.478]  I2=[4.71e-13 356.3 356.3;377 377 377;-2.438 0.173 -1.398]  nHarmo=1  Measurements=None
  Fault : powerlib/Elements/Three-Phase Fault  Commented=on  InitialStates=0  FaultA=on  FaultB=off  FaultC=off  GroundFault=on  SwitchTimes=1  External=off  SwitchStatus=NaN  FaultResistance=1e-9  GroundResistance=0.01  SnubberResistance=1e6  SnubberCapacitance=inf  Measurements=None
  Linear Transformer1 : powerlib/Elements/Linear Transformer  UNITS=pu  NominalPower=[ 150e8 60 ]  winding1=[230e3 0.002 1]  winding2=[230e3 0.002 1]  ThreeWindings=off  winding3=[3.15e+05 0.002 0.079997]  RmLm=[499.99 500]  Measurements=None  DataType=off
  Linear Transformer2 : powerlib/Elements/Linear Transformer  UNITS=pu  NominalPower=[150e8 60 ]  winding1=[230e3 0.002 1]  winding2=[230e3 0.002 1]  ThreeWindings=off  winding3=[3.15e+05 0.002 0.079997]  RmLm=[499.99 500]  Measurements=None  DataType=off
  Linear Transformer3 : powerlib/Elements/Linear Transformer  UNITS=pu  NominalPower=[ 150e8 60 ]  winding1=[230e3 0.002 1]  winding2=[230e3 0.002 1]  ThreeWindings=off  winding3=[3.15e+05 0.002 0.079997]  RmLm=[499.99 500]  Measurements=None  DataType=off
  Mimic Filter & Sampling : Subsystem
  Relay : Subsystem
  Scope : Scope  NumInputPorts=3
  Voltage Measurement Algorithm : Subsystem
  powergui : powerlib/powergui  Priority=1  SimulationMode=Discrete  SampleTime=1/1200/30  frequency=60  Iterations=50  frequencyindice=60  Pbase=100e6  ErrMax=0.0001  UnitsV=kV  UnitsW=MW  buscounter=0  FunctionMessages=off  echomessages=off  EnableUseOfTLC=off  CurrentSourceSwitches=off  DisableSnubberDevices=off  DisableRonSwitches=off  DisableVfSwitches=off  DisplayEquations=off  AutomaticDiscreteSolvers=off  SolverType=Tustin/Backward Euler (TBE)  Interpol=off  ExternalGateDelay=off  methode=off  Ts=100  x0status=blocks  SPID=on  SwTol=0  HookPort=off  NonlinearTolerance=1e-4  nMaxIteration=100  ContinueOnMaxIteration=off  RestoreLinks=warning  ResistiveCurrentMeasurement=off  Frange=[0:2:500]  Ylog=off  Xlog=on  ShowGrid=off  save=off  variable=ZData  structure=0  ZoomFFT=off  StartTime=0.0  cycles=1  DisplayStyle=1  fundamental=60  FreqAxis=off  MaxFrequency=1000  frequencyindicesteady=1  RmsSteady=1  display=off
  tag scope: Ia=global, Ib=global, Ic=global
  wires:
  Mimic Filter & Sampling/1(Ia) -> Scope/1, [Ia]
  Mimic Filter & Sampling/2(Ib) -> Scope/2, [Ib]
  Mimic Filter & Sampling/3(Ic) -> Scope/3, [Ic]
  connections:
  Distributed Parameters Line3/LConn2 -- Distributed Parameters Line1/RConn2 -- 100+j35 MVA/LConn2 -- Fault/LConn2
  Distributed Parameters Line3/LConn3 -- Distributed Parameters Line1/RConn3 -- Fault/LConn3 -- 100+j35 MVA/LConn3
  Distributed Parameters Line5/RConn1 -- Distributed Parameters Line8/LConn1 -- 90+j30 MVA/LConn1
  Distributed Parameters Line5/RConn3 -- Distributed Parameters Line8/LConn3 -- 90+j30 MVA/LConn3
  Distributed Parameters Line6/LConn1 -- Distributed Parameters Line7/LConn1 -- 125+j50 MVA/LConn1
  Distributed Parameters Line6/LConn2 -- Distributed Parameters Line7/LConn2 -- 125+j50 MVA/LConn2
  Distributed Parameters Line6/LConn3 -- Distributed Parameters Line7/LConn3 -- 125+j50 MVA/LConn3
  Distributed Parameters Line3/RConn1 -- 13.8 KV/230 KV 5.86 %Z/RConn1 -- Distributed Parameters Line8/RConn1
  Distributed Parameters Line3/RConn2 -- 13.8 KV/230 KV 5.86 %Z/RConn2 -- Distributed Parameters Line8/RConn2
  Distributed Parameters Line3/RConn3 -- 13.8 KV/230 KV 5.86 %Z/RConn3 -- Distributed Parameters Line8/RConn3
  18KV/230KV 6.25 %Z/RConn1 -- Relay/LConn1 -- Distributed Parameters Line7/RConn1
  18KV/230KV 6.25 %Z/RConn2 -- Relay/LConn2 -- Distributed Parameters Line7/RConn2
  18KV/230KV 6.25 %Z/RConn3 -- Relay/LConn3 -- Distributed Parameters Line7/RConn3
  Distributed Parameters Line5/RConn2 -- Distributed Parameters Line8/LConn2 -- 90+j30 MVA/LConn2
  Distributed Parameters Line6/RConn1 -- "16.5 KV/230 KV 5.76 %Z     "/RConn1 -- Distributed Parameters Line5/LConn1
  Distributed Parameters Line6/RConn2 -- "16.5 KV/230 KV 5.76 %Z     "/RConn2 -- Distributed Parameters Line5/LConn2
  Distributed Parameters Line6/RConn3 -- "16.5 KV/230 KV 5.76 %Z     "/RConn3 -- Distributed Parameters Line5/LConn3
  247.5 MW/RConn1 -- "16.5 KV/230 KV 5.76 %Z     "/LConn1
  247.5 MW/RConn2 -- "16.5 KV/230 KV 5.76 %Z     "/LConn2
  247.5 MW/RConn3 -- "16.5 KV/230 KV 5.76 %Z     "/LConn3
  128 MW/RConn1 -- 13.8 KV/230 KV 5.86 %Z/LConn1
  128 MW/RConn2 -- 13.8 KV/230 KV 5.86 %Z/LConn2
  128 MW/RConn3 -- 13.8 KV/230 KV 5.86 %Z/LConn3
  192 MW/RConn1 -- 18KV/230KV 6.25 %Z/LConn1
  192 MW/RConn2 -- 18KV/230KV 6.25 %Z/LConn2
  192 MW/RConn3 -- 18KV/230KV 6.25 %Z/LConn3
  Mimic Filter & Sampling/LConn1 -- Linear Transformer2/RConn1
  Mimic Filter & Sampling/LConn2 -- Linear Transformer2/RConn2
  Linear Transformer1/RConn1 -- Mimic Filter & Sampling/LConn3
  Linear Transformer1/RConn2 -- Mimic Filter & Sampling/LConn4
  Linear Transformer3/RConn1 -- Mimic Filter & Sampling/LConn5
  Linear Transformer3/RConn2 -- Mimic Filter & Sampling/LConn6
  100+j35 MVA/LConn1 -- Fault/LConn1 -- Distributed Parameters Line1/RConn1 -- Distributed Parameters Line3/LConn1
  Linear Transformer2/LConn1 -- Relay/RConn1
  Linear Transformer2/LConn2 -- Distributed Parameters Line1/LConn1
  Linear Transformer1/LConn1 -- Relay/RConn2
  Linear Transformer1/LConn2 -- Distributed Parameters Line1/LConn2
  Linear Transformer3/LConn1 -- Relay/RConn3
  Linear Transformer3/LConn2 -- Distributed Parameters Line1/LConn3

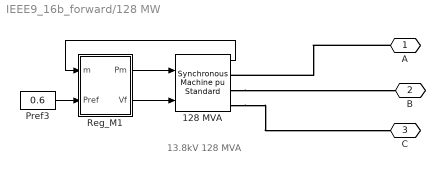
== system IEEE9_16b_forward/128 MW ==
  note: 13.8kV 128 MVA
  128 MVA : powerlib/Machines/Synchronous Machine pu Standard  PresetModel=No  MechanicalLoad=Mechanical power Pm  ShowDetailedParameters=on  RotorType=Salient-pole  Units=per unit standard parameters  MeasurementBus=off  NominalParameters="[128e6  13800   60 ]"  Reactances1=[ 31 32 33 34 35 36 37 ]  Reactances2=[ 1.305, 0.296, 0.252, 0.474, 0.243, 0.18 ]  dAxisTimeConstants=Short-circuit  qAxisTimeConstants=Open-circuit  TimeConstants1=[]  TimeConstants2=[]  TimeConstants3=[]  TimeConstants4=[]  TimeConstants5=[ 1.01, 0.053, 0.1 ]  TimeConstants6=[]  TimeConstants7=[]  TimeConstants8=[]  StatorResistance=2.8544e-3  Mechanical="[20 0  32]"  PolePairs=32  InitialConditions=[0 -74.5248 0.603223 0.603223 0.603223 5.08525 -114.915 125.085 1.10339]  SetSaturation=off  Saturation=[0.6404,0.7127,0.8441,0.9214,0.9956,1.082,1.19,1.316,1.457;0.7,0.7698,0.8872,0.9466,0.9969,1.046,1.1,1.151,1.201]  LoadFlowParameters=[1 500000000 0 0 0]  TsPowergui=0  TsBlock=-1  IterativeModel=Trapezoidal non iterative  IterativeDiscreteModel=Trapezoidal non iterative  BusType=PV  Pref=0.6*128e6  Qref=0  Qmin=-Inf  Qmax=Inf  PLF=0  QLF=0
      settings: AttributesFormatString=\n\n
  Pref3 : Constant  Value=0.6
  Reg_M1 : Subsystem
  A : PMIOPort  Side=Right
  B : PMIOPort  Port=2  Side=Right
  C : PMIOPort  Port=3  Side=Right
  wires:
  Reg_M1/1(Pm) -> 128 MVA/1
  Reg_M1/2(Vf) -> 128 MVA/2
  Pref3/1 -> Reg_M1/2(Pref)
  128 MVA/1 -> Reg_M1/1(m)
  connections:
  A/RConn1 -- 128 MVA/RConn1
  128 MVA/RConn2 -- B/RConn1
  128 MVA/RConn3 -- C/RConn1
